simulink model "SampleTime1"  (R2015a)
settings: Solver=FixedStepDiscrete  SolverMode=SingleTasking  StartTime=0.0  StopTime=10.0  RelTol=1e-3
undefined symbols (not defined in the file): sldvsubsys
settings Model: CovMetricSettings=dwe  CovHtmlReporting=off  covSaveCumulativeToWorkspaceVar=off  CovSaveSingleToWorkspaceVar=off  CovExternalEMLEnable=on  Creator=hbourbou  LastModifiedBy=hbourbou
settings DataIOCC: LimitDataPoints=off  SaveFormat=Dataset
settings DebuggingCC: SFUnexpectedBacktrackingDiag=error  SFNoUnconditionalDefaultTransitionDiag=error
settings HardwareCC: ProdBitPerPointer=64  ProdLargestAtomicFloat=Float  ProdIntDivRoundTo=Zero  ProdEndianess=LittleEndian  ProdHWDeviceType=Specified
settings ModelReferenceCC: PropagateSignalLabelsOutOfModel=on
settings GRTTargetCC: TargetLangStandard=C99 (ISO)  GeneratePreprocessorConditionals=Use local settings

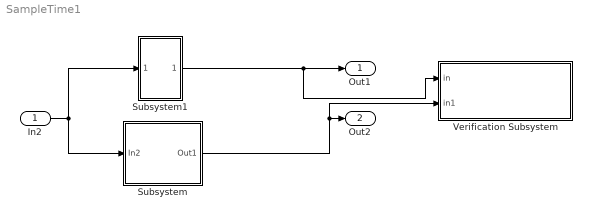
== system SampleTime1 ==
  In2 : Inport  OutDataTypeStr=int8  SampleTime=1
  Subsystem : Subsystem
  Subsystem1 : Subsystem
  Verification Subsystem : Subsystem  Tag=VerificationSubsystem  DisableCoverage=on  LoadFcn=sldvsubsys('check')  TreatAsAtomicUnit=on  SimViewingDevice=on  mask(VerificationSubsystem){}
      mask init:
      | sldvsubsys('maskInit');
      settings: CopyFcn=sldvsubsys('copy');  OpenFcn=open_system(gcb,'force');
      settings: PreSaveFcn=|
      | set_param(gcb,'SimViewingDevice','on');
      | sldvsubsys('check');
      mask Help: helpview(fullfile(docroot,'toolbox','sldv','sldv.map'),'verificationsubsystem')
      mask Display: image(imread('sldvicon_versubsys.png','BackGroundColor',[1 1 1]),'center');
  Out1 : Outport
  Out2 : Outport  Port=2
  wires:
  Subsystem/1(Out1) -> Verification Subsystem/2(in1), Out2/1
  Subsystem1/1(Out1) -> Verification Subsystem/1(in), Out1/1
  In2/1 -> Subsystem1/1(In1), Subsystem/1(In2)

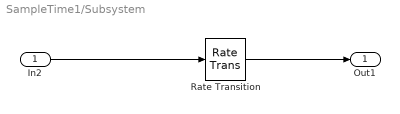
== system SampleTime1/Subsystem ==
  In2 : Inport  OutDataTypeStr=int8  SampleTime=1
  Rate Transition : RateTransition  Integrity=off  OutPortSampleTime=2
  Out1 : Outport
  wires:
  In2/1 -> Rate Transition/1
  Rate Transition/1 -> Out1/1

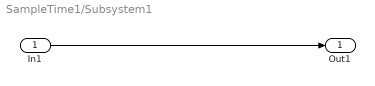
== system SampleTime1/Subsystem1 ==
  In1 : Inport  OutDataTypeStr=int8  SampleTime=2
  Out1 : Outport
  wires:
  In1/1 -> Out1/1

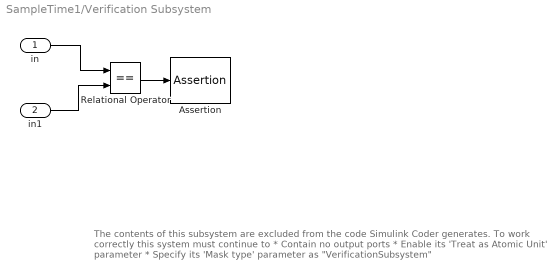
== system SampleTime1/Verification Subsystem ==
  note: The contents of this subsystem are excluded from the code Simulink Coder
      | generates.
      |
      | To work correctly this system must continue to
      | * Contain no output ports
      | * Enable its 'Treat as Atomic Unit' parameter
      | * Specify its 'Mask type' parameter as "VerificationSubsystem"
  in : Inport
  in1 : Inport  Port=2
  Assertion : Assertion
  Relational Operator : RelationalOperator  Operator===  OutDataTypeStr=boolean
  wires:
  in/1 -> Relational Operator/1
  in1/1 -> Relational Operator/2
  Relational Operator/1 -> Assertion/1
